simulink model "testing_angles"  (R2013a)
settings: Solver=ode3  StartTime=0.0  StopTime=10.0  RelTol=1e-3
model workspace (MATLAB code in the model file):
  | % ________________________________________
  | %
  | %                HYL DESCRIPTION PARAMETERS
  | %________________________________________
  | 
  | % ---- Leg data ------
  | 
  | m1 = 1.772;              % Kg - Upper leg mass
  | m2 = 0.808;              % Kg - Lower leg mass
  | M = 3.982;                % Kg - Base mass
  | P_01 = 0.08;             % m - distance P0-P1
  | P_12 = 0.350;           % m - distance P1-P2
  | P_23 = 0.330;           % m - distance P2-P3
  | FR = 0.02;                 % m - foot radius
  | P1m1 = 0.164;           % m - distance P1-Pm1
  | P2m2 = 0.122;           % m - distance P2-Pm2
  | I1zz = 0.0713;           % kg·m2 - Inertia upper leg
  | I2zz = 0.0218;           % kg·m2 - Inertia lower leg
  | em1 = deg2rad(7.9);  % rad
  | em2 = deg2rad(0);     % rad
  | g  = 9.810;                 % m/s2 - gravity
  | 
  | % ----- Lever Arm Parameters -----
  | 
  | % Hip joint
  | a1   = 0.3219;             % m
  | b1   = 0.045;               % m
  | e11 = deg2rad(6.24); % rad
  | e12 = deg2rad(0);      % rad
  | 
  | % Knee joint
  | a2 = 0.3218;               % m
  | b2 = 0.045;                 % m
  | e21 = deg2rad(8.04);  % rad
  | e22 = deg2rad(6);       % rad
  | 
  | % ----- Limit Angles --------
  | 
  | % Initial conditions
  | q0_0 = 1;                           % m - height of the floating base
  | q1_0 = deg2rad(45);         % rad - HFE angle
  | q2_0 = deg2rad(-90);        % rad - KFE angle
  | 
  | % Max angle limits
  | q1Max = deg2rad(70);       % rad
  | q2Max = deg2rad(-20);      % rad
  | 
  | % Min angle limits
  | q1Min = deg2rad(-50);        % rad
  | q2Min = deg2rad(-140);      % rad
  | q0Min = P_01+P_12*cos(q1Min)+P_23*cos(q1Min+q2Min)+FR;     % m
undefined symbols (not defined in the file): sigbuilder_block
settings Model: Creator=Toshiba  LastModifiedBy=Toshiba

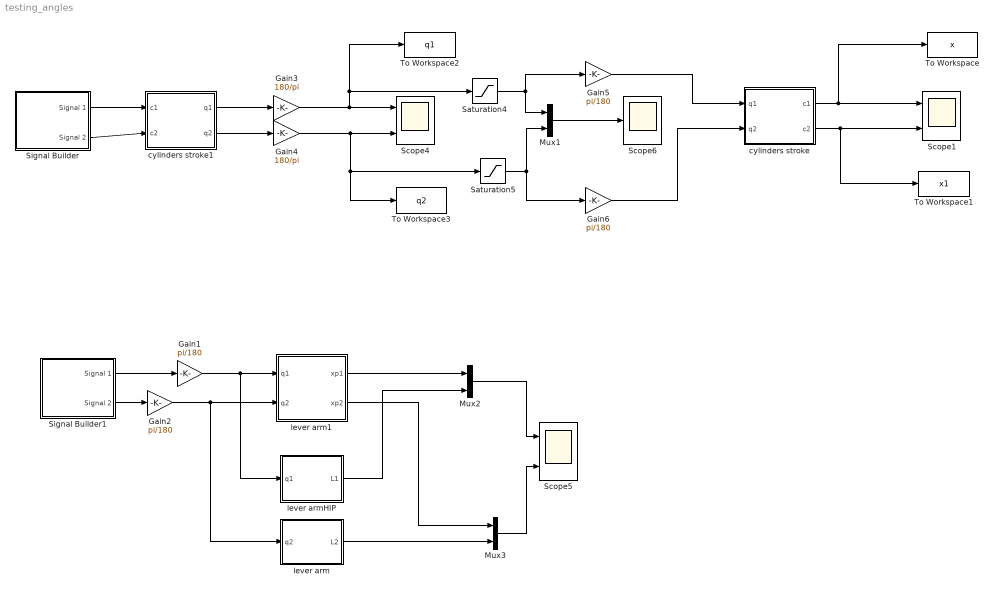
== system testing_angles ==
  Gain{1..2,5..6} (4 alike) : Gain  Gain=pi/180
  Gain3 : Gain  Gain=180/pi
  Gain4 : Gain  Gain=180/pi
  Mux1 : Mux  Inputs=2
  Mux2 : Mux  Inputs=2
  Mux3 : Mux  Inputs=2
  Saturation4 : Saturate  UpperLimit=70  LowerLimit=-50
  Saturation5 : Saturate  UpperLimit=-20  LowerLimit=-140
  Scope1 : Scope  NumInputPorts=2
      settings: YMin=0.196~-5  YMax=0.211~5
  Scope4 : Scope  NumInputPorts=2
      settings: YMin=0.196~-5  YMax=0.211~5  SaveName=ScopeData4
  Scope5 : Scope  NumInputPorts=2
      settings: YMin=0.196~-5  YMax=0.211~5  SaveName=ScopeData3
  Scope6 : Scope
      settings: YMin=0.196  YMax=0.211  SaveName=ScopeData6
  Signal Builder : Subsystem  Tag=STV Subsys  LoadFcn=sigbuilder_block('load');  StartFcn=sigbuilder_block('start');  StopFcn=sigbuilder_block('stop');  ClipboardFcn=sigbuilder_block('clipboard');  mask(Sigbuilder block){}
      mask help: Simulink:masks:SigbuilderBlock_MD
      mask init:
      | if ~strcmp(get_param(bdroot(gcbh),'SimulationStatus'),'stopped') tuvar = sigbuilder_block('maskInit'); end
      settings: CopyFcn=sigbuilder_block('copy');  DeleteFcn=sigbuilder_block('delete');  ModelCloseFcn=sigbuilder_block('modelClose');  PreSaveFcn=sigbuilder_block('preSave');  PauseFcn=sigbuilder_block('pause');  ContinueFcn=sigbuilder_block('continue');  NameChangeFcn=sigbuilder_block('namechange');  OpenFcn=sigbuilder_block('open',[437.25 117.75 550.5 394.5 ]);  CloseFcn=sigbuilder_block('close');
      mask Display: plot(0, 0, 100, 100,[2, 2, 32, 32, 2], [68, 8, 8, 68, 68],[32, 2], [38, 38], [32, 19, 2],[53, 60, 44], [32, 17, 17, 2],[16, 16, 31, 31]);txt = getActiveGroup(gcbh);text(2, 100, txt,'verticalAlignment', 'top');
  Signal Builder1 : Subsystem  Tag=STV Subsys  LoadFcn=sigbuilder_block('load');  StartFcn=sigbuilder_block('start');  StopFcn=sigbuilder_block('stop');  ClipboardFcn=sigbuilder_block('clipboard');  mask(Sigbuilder block){}
      mask help: Simulink:masks:SigbuilderBlock_MD
      mask init:
      | if ~strcmp(get_param(bdroot(gcbh),'SimulationStatus'),'stopped') tuvar = sigbuilder_block('maskInit'); end
      settings: CopyFcn=sigbuilder_block('copy');  DeleteFcn=sigbuilder_block('delete');  ModelCloseFcn=sigbuilder_block('modelClose');  PreSaveFcn=sigbuilder_block('preSave');  PauseFcn=sigbuilder_block('pause');  ContinueFcn=sigbuilder_block('continue');  NameChangeFcn=sigbuilder_block('namechange');  OpenFcn=sigbuilder_block('open',[437.25 117.75 550.5 394.5 ]);  CloseFcn=sigbuilder_block('close');
      mask Display: plot(0, 0, 100, 100,[2, 2, 32, 32, 2], [68, 8, 8, 68, 68],[32, 2], [38, 38], [32, 19, 2],[53, 60, 44], [32, 17, 17, 2],[16, 16, 31, 31]);txt = getActiveGroup(gcbh);text(2, 100, txt,'verticalAlignment', 'top');
  To Workspace : ToWorkspace  VariableName=x  SampleTime=-1
  To Workspace1 : ToWorkspace  VariableName=x1  SampleTime=-1
  To Workspace2 : ToWorkspace  VariableName=q1  SampleTime=-1
  To Workspace3 : ToWorkspace  VariableName=q2  SampleTime=-1
  cylinders stroke : MATLAB Function  TreatAsAtomicUnit=on
  cylinders stroke1 : MATLAB Function  TreatAsAtomicUnit=on
  lever arm : MATLAB Function  TreatAsAtomicUnit=on
  lever arm1 : MATLAB Function  TreatAsAtomicUnit=on
  lever armHIP : MATLAB Function  TreatAsAtomicUnit=on
  wires:
  cylinders stroke1/2(q2) -> Gain4/1
  cylinders stroke1/1(q1) -> Gain3/1
  Gain3/1 -> Scope4/1, To Workspace2/1, Saturation4/1
  Gain4/1 -> Scope4/2, Saturation5/1, To Workspace3/1
  Saturation4/1 -> Mux1/1, Gain5/1
  Saturation5/1 -> Gain6/1, Mux1/2
  Mux1/1 -> Scope6/1
  cylinders stroke/2(c2) -> Scope1/2, To Workspace1/1
  cylinders stroke/1(c1) -> Scope1/1, To Workspace/1
  Signal Builder/1(Signal 1) -> cylinders stroke1/1(c1)
  Signal Builder/2(Signal 2) -> cylinders stroke1/2(c2)
  Gain5/1 -> cylinders stroke/1(q1)
  Gain6/1 -> cylinders stroke/2(q2)
  Signal Builder1/2(Signal 2) -> Gain2/1
  Signal Builder1/1(Signal 1) -> Gain1/1
  lever arm1/1(xp1) -> Mux2/1
  lever arm1/2(xp2) -> Mux3/1
  Gain1/1 -> lever armHIP/1(q1), lever arm1/1(q1)
  Gain2/1 -> lever arm/1(q2), lever arm1/2(q2)
  lever armHIP/1(L1) -> Mux2/2
  Mux2/1 -> Scope5/1
  Mux3/1 -> Scope5/2
  lever arm/1(L2) -> Mux3/2

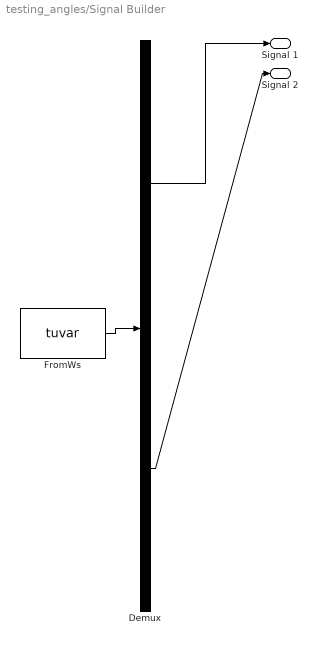
== system testing_angles/Signal Builder ==
  Demux : Demux  Tag=STV Demux  Outputs=2
  FromWs : FromWorkspace  Tag=STV FromWs  VariableName=tuvar  SampleTime=0
      SigBuilderData=|
      | common.afterFinalStr = 'Extrapolate'
      | common.sampleTime = 0
      | dataSet(1).timeRange = [0 10]
      | dataSet(1).name = 'Group 1'
      | dataSet(2).timeRange = [0 10]
      | dataSet(2).name = 'Group 2'
      | sbobj.Groups(1).Name = 'Group 1'
      | sbobj.Groups(1).Signals(1).Name = 'Signal 1'
      | sbobj.Groups(1).Signals(1).XData = [0 4 5 7 8 10]
      | sbobj.Groups(1).Signals(1).YData = [0.28 0.28 0.36 0.36 0.28 0.28]
      | sbobj.Groups(1).Signals(2).Name = 'Signal 2'
      | sbobj.Groups(1).Signals(2).XData = [0 4 5 7 8 10]
      | sbobj.Groups(1).Signals(2).YData = [0.28 0.28 0.36 0.36 0.28 0.28]
      | sbobj.Groups(2).Name = 'Group 2'
      | sbobj.Groups(2).Signals(1).Name = 'Signal 1'
      | sbobj.Groups(2).Signals(1).XData = [0 4 5 7 8 10]
      | sbobj.Groups(2).Signals(1).YData = [0.28 0.28 0.36 0.36 0.28 0.28]
      | sbobj.Groups(2).Signals(2).Name = 'Signal 2'
      | sbobj.Groups(2).Signals(2).XData = [0 10]
      | sbobj.Groups(2).Signals(2).YData = [0 0]
  Signal 1 : Outport  Tag=STV Outport
  Signal 2 : Outport  Tag=STV Outport  Port=2
  wires:
  Demux/1 -> Signal 1/1
  FromWs/1 -> Demux/1
  Demux/2 -> Signal 2/1

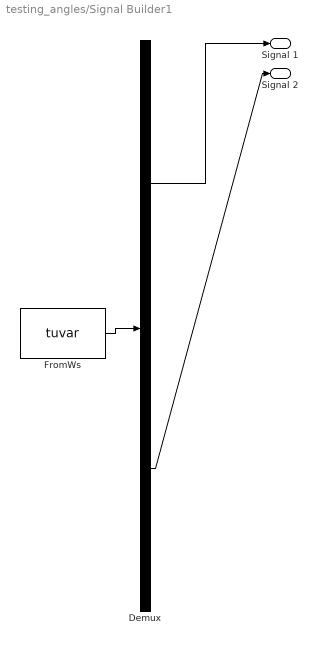
== system testing_angles/Signal Builder1 ==
  Demux : Demux  Tag=STV Demux  Outputs=2
  FromWs : FromWorkspace  Tag=STV FromWs  VariableName=tuvar  SampleTime=0
      SigBuilderData=|
      | common.afterFinalStr = 'Extrapolate'
      | common.sampleTime = 0
      | dataSet(1).timeRange = [0 10]
      | dataSet(1).name = 'Group 1'
      | dataSet(2).timeRange = [0 10]
      | dataSet(2).name = 'Group 2'
      | sbobj.Groups(1).Name = 'Group 1'
      | sbobj.Groups(1).Signals(1).Name = 'Signal 1'
      | sbobj.Groups(1).Signals(1).XData = [0 4 5 7 8 10]
      | sbobj.Groups(1).Signals(1).YData = [-50 -50 70 70 -50 -50]
      | sbobj.Groups(1).Signals(2).Name = 'Signal 2'
      | sbobj.Groups(1).Signals(2).XData = [0 4 5 7 8 10]
      | sbobj.Groups(1).Signals(2).YData = [-140 -140 -20 -20 -140 -140]
      | sbobj.Groups(2).Name = 'Group 2'
      | sbobj.Groups(2).Signals(1).Name = 'Signal 1'
      | sbobj.Groups(2).Signals(1).XData = [0 4 5 7 8 10]
      | sbobj.Groups(2).Signals(1).YData = [0.28 0.28 0.36 0.36 0.28 0.28]
      | sbobj.Groups(2).Signals(2).Name = 'Signal 2'
      | sbobj.Groups(2).Signals(2).XData = [0 10]
      | sbobj.Groups(2).Signals(2).YData = [0 0]
  Signal 1 : Outport  Tag=STV Outport
  Signal 2 : Outport  Tag=STV Outport  Port=2
  wires:
  Demux/2 -> Signal 2/1
  FromWs/1 -> Demux/1
  Demux/1 -> Signal 1/1

== matlab function testing_angles/cylinders stroke1 ==
  data: a1 parameter; q1 output; b1 parameter; e11 parameter; e12 parameter; a2 parameter; b2 parameter; e21 parameter; e22 parameter; c1 input; q2 output; c2 input
function [q1,q2] = fcn(a1,b1,e11,e12,a2,b2,e21,e22,c1,c2)
%#codegen

%Hip
ang1 = acos(((a1^2+b1^2)-c1^2)/(2*a1*b1));
q1 = pi/2 - ang1 + e11 - e12; 

%Knee
ang2 = acos(((a2^2+b2^2)-c2^2)/(2*a2*b2));
q2 = - pi + ang2 + e21 + e22;

== matlab function testing_angles/lever arm1 ==
  data: a1 parameter; xp1 output; b1 parameter; e11 parameter; e12 parameter; a2 parameter; b2 parameter; e21 parameter; e22 parameter; q1 input; q2 input; xp2 output
function [xp1,xp2] = fcn(a1,b1,e11,e12,a2,b2,e21,e22,q1,q2)
%#codegen

%Hip
ang1 = pi/2 - q1 + e11 - e12; 
c1 = sqrt(a1^2 + b1^2 - 2*a1*b1*cos(ang1));

%Knee
ang2 = pi + q2 - e21 - e22;
c2 = sqrt(a2^2 + b2^2 - 2*a2*b2*cos(ang2));

Lcyl = 0.281; % Total length of the cylinder when its rod is totally retracted

xp1 = c1-Lcyl;
xp2 = c2-Lcyl;

== matlab function testing_angles/lever arm ==
  data: a2 parameter; L2 output; b2 parameter; e21 parameter; e22 parameter; q2 input
function L2 = fcn(a2,b2,e21,e22,q2)
%#codegen

ang2 = pi + q2 - e21 - e22;
c2 = sqrt(a2^2 + b2^2 - 2*a2*b2*cos(ang2));
L2 = a2*sin(acos((a2^2+c2^2-b2^2)/(2*a2*c2)));

== matlab function testing_angles/lever armHIP ==
  data: a1 parameter; L1 output; b1 parameter; e11 parameter; e12 parameter; q1 input
function L1 = fcn(a1,b1,e11,e12,q1)
%#codegen

ang1 = pi/2 - q1 + e11 - e12;
c1 = sqrt(a1^2 + b1^2 - 2*a1*b1*cos(ang1));
L1 = a1*sin(acos((a1^2+c1^2-b1^2)/(2*a1*c1)));

== matlab function testing_angles/cylinders stroke ==
  data: a1 parameter; c1 output; b1 parameter; e11 parameter; e12 parameter; a2 parameter; b2 parameter; e21 parameter; e22 parameter; q1 input; c2 output; q2 input
function [c1,c2] = fcn(a1,b1,e11,e12,a2,b2,e21,e22,q1, q2)
%#codegen

%Hip
ang1 = pi/2 - q1 + e11 - e12; 
c1 = sqrt(a1^2 + b1^2 - 2*a1*b1*cos(ang1));

%Knee
ang2 = pi + q2 - e21 - e22;
c2 = sqrt(a2^2 + b2^2 - 2*a2*b2*cos(ang2));
